simulink model "Open_loop_robot"  (R2024b)
settings: Solver=ode45  StartTime=0.0  StopTime=TF  MaxStep=1e-2  RelTol=1e-3  EnableMultiTasking=on
values from neighbouring files (symbols this model uses):
  amplitud = [15 15 20]    [robot_definition.m]    (also in sinusoidal_torque_inputs.m)
  offset = [0 20 0]    [robot_definition.m]    (also in sinusoidal_torque_inputs.m)
  Tm = 0.001    [controlled_robot_def_Nested.m]    (also in controlled_robot_def_PD.m; controlled_robot_def_PID.m = 0.01; controlled_robot_def_ctorque.m = 0.01; controlled_robot_def_freedfwrd.m = 0.01)
libraries: roblocks x1
settings Model: Creator=gbejarano  LastModifiedBy=pcarn
settings SolverCC: AlgebraicLoopSolver=TrustRegion
settings DataIOCC: LimitDataPoints=on  SaveFormat=Array  SignalLoggingSaveFormat=ModelDataLogs  ReturnWorkspaceOutputs=off
settings OptimizationCC: InitFltsAndDblsToZero=on  LifeSpan=inf
settings DebuggingCC: SaveWithParameterizedLinksMsg=none  UnderspecifiedInitializationDetection=Classic  MergeDetectMultiDrivingBlocksExec=none  SignalResolutionControl=TryResolveAllWithWarning  MultiTaskDSMMsg=warning  MultiTaskCondExecSysMsg=none  UnconnectedInputMsg=warning  UnconnectedOutputMsg=warning  UnconnectedLineMsg=warning  SFUnexpectedBacktrackingDiag=warning  SFNoUnconditionalDefaultTransitionDiag=warning  SFExecutionAtInitializationDiag=none  ArithmeticOperatorsInVariantConditions=warning
settings HardwareCC: ProdBitPerPointer=32  ProdBitPerSizeT=32  ProdBitPerPtrDiffT=32  ProdLargestAtomicFloat=None  ProdIntDivRoundTo=Undefined  ProdEndianess=Unspecified  ProdWordSize=32  ProdHWDeviceType=32-bit Generic
settings ModelReferenceCC: EnableRefExpFcnMdlSchedulingChecks=on  PropagateSignalLabelsOutOfModel=off
settings SFSimCC: CustomCodeUndefinedFunction=UseInterfaceOnly
settings RTWCC: GPUComputeCapability=3.5
settings CodeAppCC: StateflowObjectComments=on
settings GRTTargetCC: TargetFcnLib=ansi_tfl_tmw.mat  TargetLangStandard=C89/C90 (ANSI)  CombineOutputUpdateFcns=off  GRTInterface=on
settings ConfigComp: CovMetricSettings=dw  CovSaveCumulativeToWorkspaceVar=on  CovSaveSingleToWorkspaceVar=on

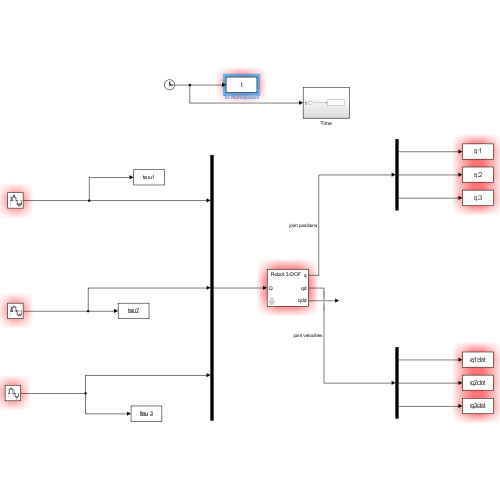
[thumbnail: Simulink's stored preview of the top-level diagram]
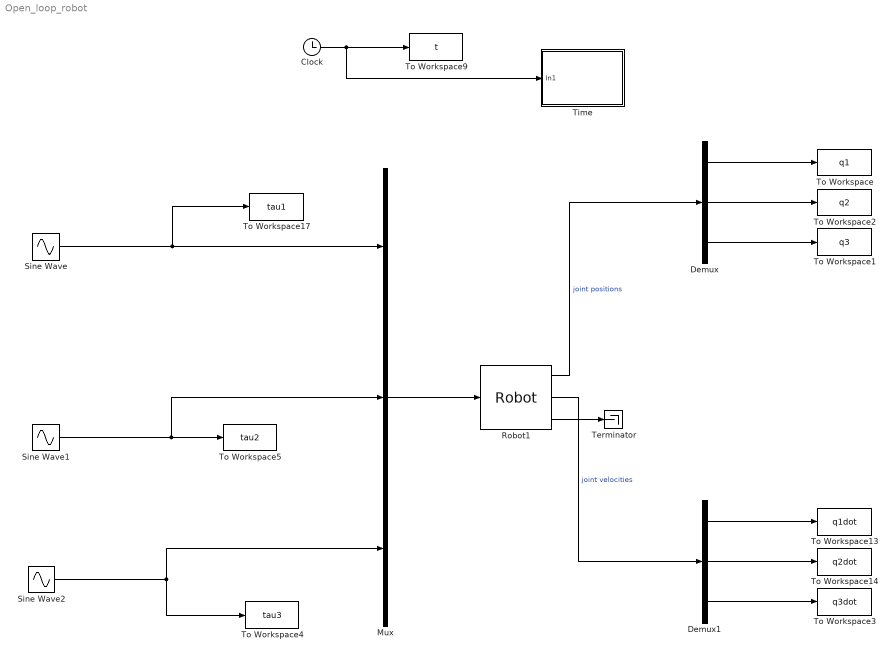
== system Open_loop_robot ==
  Clock : Clock
  Demux : Demux  Outputs=3
  Demux1 : Demux  Outputs=3
  Mux : Mux  Inputs=3
  Robot1 : roblocks/Arm/Robot  robot=robot_3dof  q0=qi
  Sine Wave : Sin  Amplitude=amplitud(1)  Bias=offset(1)  SampleTime=Tm
  Sine Wave1 : Sin  Amplitude=amplitud(2)  Bias=offset(2)  SampleTime=Tm
  Sine Wave2 : Sin  Amplitude=amplitud(3)  Bias=offset(3)  SampleTime=Tm
  Terminator : Terminator
  "Time " : Subsystem
  To Workspace : ToWorkspace  VariableName=q1  SampleTime=Tm
  To Workspace1 : ToWorkspace  VariableName=q3  SampleTime=Tm
  To Workspace13 : ToWorkspace  VariableName=q1dot  SampleTime=Tm
  To Workspace14 : ToWorkspace  VariableName=q2dot  SampleTime=Tm
  To Workspace17 : ToWorkspace  VariableName=tau1  SampleTime=-1
  To Workspace2 : ToWorkspace  VariableName=q2  SampleTime=Tm
  To Workspace3 : ToWorkspace  VariableName=q3dot  SampleTime=Tm
  To Workspace4 : ToWorkspace  VariableName=tau3  SampleTime=-1
  To Workspace5 : ToWorkspace  VariableName=tau2  SampleTime=-1
  To Workspace9 : ToWorkspace  VariableName=t  SampleTime=Tm
  wires:
  Clock/1 -> "Time "/1(In1), To Workspace9/1
  Sine Wave1/1 -> Mux/2, To Workspace5/1
  Demux/2 -> To Workspace2/1
  Sine Wave/1 -> Mux/1, To Workspace17/1
  Demux1/2 -> To Workspace14/1
  Demux1/1 -> To Workspace13/1
  Demux/1 -> To Workspace/1
  Mux/1 -> Robot1/1
  Robot1/1 -> Demux/1  "joint positions"
  Robot1/2 -> Demux1/1  "joint velocities"
  Robot1/3 -> Terminator/1
  Demux/3 -> To Workspace1/1
  Demux1/3 -> To Workspace3/1
  Sine Wave2/1 -> To Workspace4/1, Mux/3

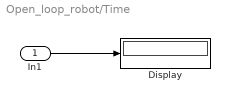
== system Open_loop_robot/Time  ==
  In1 : Inport
  Display : Display
  wires:
  In1/1 -> Display/1
